simulink model "simOrbit"  (R2017b)
settings: Solver=VariableStepAuto  StartTime=0.0  StopTime=10  RelTol=1e-6
values from neighbouring files (symbols this model uses):
  const = -39.4887    [orbitatierra2.m]
  IP = 1.016714    [orbitatierra2.m]
  IV = 6.1798    [orbitatierra2.m]
settings Model: Creator=luisr  LastModifiedBy=luisr

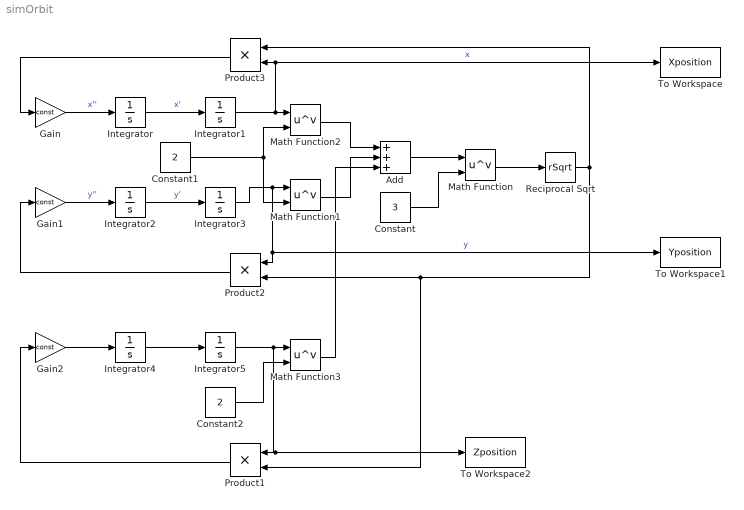
== system simOrbit ==
  Add : Sum  Inputs=+++
  Constant : Constant  Value=3
  Constant1 : Constant  Value=2
  Constant2 : Constant  Value=2
  Gain : Gain  Gain=const
  Gain1 : Gain  Gain=const
  Gain2 : Gain  Gain=const
  Integrator{,3..5} (4 alike) : Integrator
  Integrator1 : Integrator  InitialCondition=IP
  Integrator2 : Integrator  InitialCondition=IV
  Math Function{,1..3} (4 alike) : Math  Operator=pow  SaturateOnIntegerOverflow=on
  Product1 : Product
  Product2 : Product
  Product3 : Product
  Reciprocal Sqrt : Sqrt  Operator=rSqrt  SaturateOnIntegerOverflow=on
  To Workspace : ToWorkspace  VariableName=Xposition  SampleTime=-1
  To Workspace1 : ToWorkspace  VariableName=Yposition  SampleTime=-1
  To Workspace2 : ToWorkspace  VariableName=Zposition  SampleTime=-1
  wires:
  Integrator/1 -> Integrator1/1  "x'"
  Integrator2/1 -> Integrator3/1  "y'"
  Gain/1 -> Integrator/1  "x''"
  Gain1/1 -> Integrator2/1  "y''"
  Integrator1/1 -> Math Function2/1, To Workspace/1, Product3/2  "x"
  Math Function2/1 -> Add/1
  Math Function1/1 -> Add/2
  Add/1 -> Math Function/1
  Constant/1 -> Math Function/2
  Math Function/1 -> Reciprocal Sqrt/1
  Reciprocal Sqrt/1 -> Product1/2, Product2/2, Product3/1
  Product2/1 -> Gain1/1
  Product3/1 -> Gain/1
  Constant1/1 -> Math Function1/2, Math Function2/2
  Integrator3/1 -> To Workspace1/1, Product2/1, Math Function1/1  "y"
  Gain2/1 -> Integrator4/1
  Integrator4/1 -> Integrator5/1
  Integrator5/1 -> To Workspace2/1, Product1/1, Math Function3/1
  Constant2/1 -> Math Function3/2
  Product1/1 -> Gain2/1
  Math Function3/1 -> Add/3
